simulink model "malhaabertacarrin"  (R2024b)
settings: Solver=VariableStepAuto  StartTime=0.0  StopTime=100  RelTol=1e-3
values from neighbouring files (symbols this model uses):
  alpha = 0    [carrin.m]    (also in vehicle_longitudinal_openloop.m)
  b = (fmax - c*vmax^2)/vmax    (= 15.4629644943)    [carrin.m]    (also in vehicle_longitudinal_openloop.m)
  c = 0.5*rho*A*cd    (= 0.404028)    [carrin.m]    (also in vehicle_longitudinal_openloop.m)
  fmax = pmax/vmax    (= 2364.54697674)    [carrin.m]    (also in vehicle_longitudinal_openloop.m)
  g = 9.82    [carrin.m]    (also in vehicle_longitudinal_openloop.m)
  m = 1322    [carrin.m]    (also in vehicle_longitudinal_openloop.m)
settings Model: Creator=Gustavo  LastModifiedBy=Gustavo

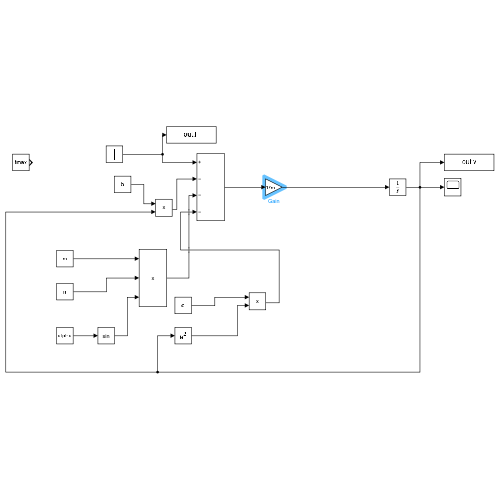
[thumbnail: Simulink's stored preview of the top-level diagram]
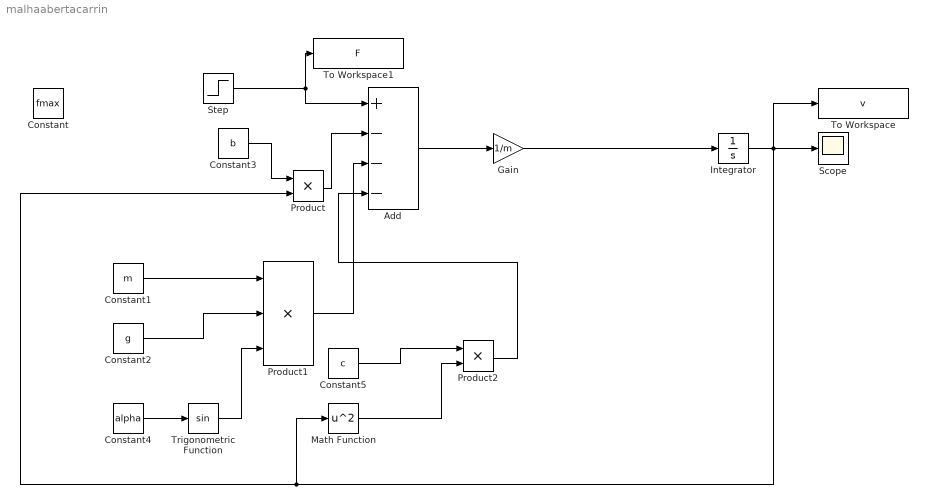
== system malhaabertacarrin ==
  Add : Sum  Inputs=+---
  Constant : Constant  Value=fmax
  Constant1 : Constant  Value=m
  Constant2 : Constant  Value=g
  Constant3 : Constant  Value=b
  Constant4 : Constant  Value=alpha
  Constant5 : Constant  Value=c
  Gain : Gain  Gain=1/m
  Integrator : Integrator
  Math Function : Math  Operator=square
  Product : Product
  Product1 : Product  Inputs=3
  Product2 : Product
  Scope : Scope
  Step : Step  After=fmax  SampleTime=0
  To Workspace : ToWorkspace  VariableName=v  SaveFormat=Timeseries  SampleTime=-1
  To Workspace1 : ToWorkspace  VariableName=F  SaveFormat=Timeseries  SampleTime=-1
  Trigonometric Function : Trigonometry
  wires:
  Add/1 -> Gain/1
  Gain/1 -> Integrator/1
  Product/1 -> Add/2
  Constant3/1 -> Product/1
  Constant1/1 -> Product1/1
  Constant2/1 -> Product1/2
  Constant4/1 -> Trigonometric Function/1
  Trigonometric Function/1 -> Product1/3
  Product1/1 -> Add/3
  Constant5/1 -> Product2/1
  Product2/1 -> Add/4
  Math Function/1 -> Product2/2
  Integrator/1 -> Math Function/1, Product/2, Scope/1, To Workspace/1
  Step/1 -> Add/1, To Workspace1/1
